simulink model "StateSpacePP_simulation"  (R2025b)
settings: Solver=FixedStepAuto  StartTime=0.0  StopTime=10.0  FixedStep=0.01  RelTol=1e-3
values from neighbouring files (symbols this model uses):
  C = [0, 1]    [PPwithStateSpace.m]
  K_1 = place(A, B, [p1 p2])    [PPwithStateSpace.m]
  K_2 = -1 / (C * inv(A_m) * B)    [PPwithStateSpace.m]
settings Model: Creator=drbha  LastModifiedBy=drbha

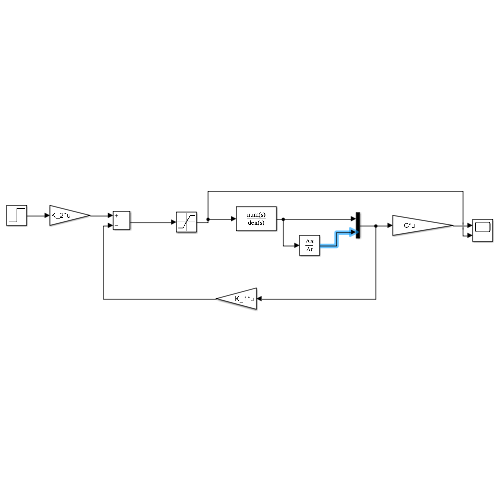
[thumbnail: Simulink's stored preview of the top-level diagram]
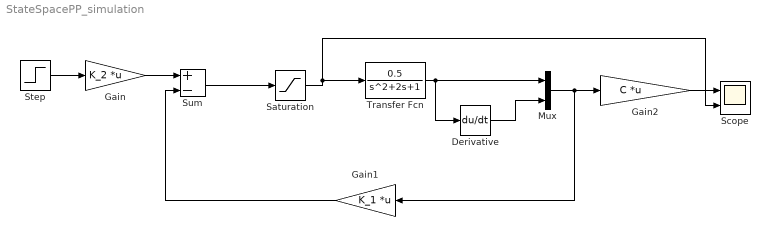
== system StateSpacePP_simulation ==
  Derivative : Derivative
  Gain : Gain  Gain=K_2  Multiplication=Matrix(K*u)
  Gain1 : Gain  Gain=K_1  Multiplication=Matrix(K*u)
  Gain2 : Gain  Gain=C  Multiplication=Matrix(K*u)
  Mux : Mux  Inputs=2
  Saturation : Saturate  UpperLimit=100  LowerLimit=0
  Scope : Scope  NumInputPorts=2
      settings: ActiveDisplayYMinimum=-1.0332661290322562  ActiveDisplayYMaximum=33.366935483870961
  Step : Step  Time=0  After=20  SampleTime=0
  Sum : Sum  Inputs=+-
  Transfer Fcn : TransferFcn  Numerator=0.5
  wires:
  Step/1 -> Gain/1
  Transfer Fcn/1 -> Mux/1, Derivative/1
  Derivative/1 -> Mux/2
  Mux/1 -> Gain2/1, Gain1/1
  Gain1/1 -> Sum/2
  Gain2/1 -> Scope/1
  Saturation/1 -> Scope/2, Transfer Fcn/1
  Gain/1 -> Sum/1
  Sum/1 -> Saturation/1
